simulink model "Sistema_LTI"  (R2016a)
settings: Solver=ode15s  StartTime=0.0  StopTime=5  RelTol=1e-3
PreLoadFcn:
  | parametros
values from neighbouring files (symbols this model uses):
  beq = (bm+bl/r^2)    (= 1.5637748692e-05)    [parametros.m]    (also in planificador_de_trayectoria.m)
  Jeq = (Jm+Jl/r^2)    (= 6.92649215207e-06)    [parametros.m]    (also in planificador_de_trayectoria.m)
  lambda_m = 0.01546    [parametros.m]
  Lq = 5.8e-3    (= 0.0058)    [parametros.m]
  Pp = 3    [parametros.m]
  r = 314.3008    [parametros.m]    (also in planificador_de_trayectoria.m)
  Rs = 1.02    [parametros.m]
settings Model: Creator=Jere  LastModifiedBy=Jere

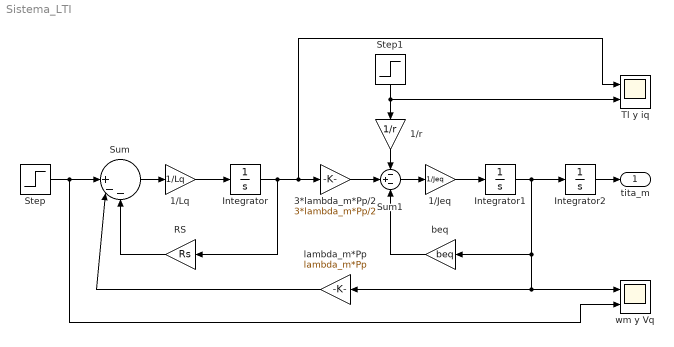
== system Sistema_LTI ==
  1/Jeq : Gain  Gain=1/Jeq
  1/Lq : Gain  Gain=1/Lq
  1/r : Gain  Gain=1/r
  3*lambda_m*Pp/2 : Gain  Gain=3*lambda_m*Pp/2
  Integrator : Integrator
  Integrator1 : Integrator
  Integrator2 : Integrator
  RS : Gain  Gain=Rs
  Step : Step  Time=0.1  After=19.596  SampleTime=0
  Step1 : Step  Time=0.3  After=1.57  SampleTime=0
  Sum : Sum  Inputs=||+--
  Sum1 : Sum  Inputs=-+-
  Tl y iq : Scope  NumInputPorts=2
  beq : Gain  Gain=beq
  lambda_m*Pp : Gain  Gain=lambda_m*Pp
  wm y Vq : Scope  NumInputPorts=2
  tita_m : Outport
  wires:
  Integrator/1 -> RS/1, Tl y iq/1, 3*lambda_m*Pp/2/1
  Integrator1/1 -> wm y Vq/1, lambda_m*Pp/1, beq/1, Integrator2/1
  Sum1/1 -> 1/Jeq/1
  1/r/1 -> Sum1/1
  3*lambda_m*Pp/2/1 -> Sum1/2
  RS/1 -> Sum/3
  Sum/1 -> 1/Lq/1
  1/Lq/1 -> Integrator/1
  beq/1 -> Sum1/3
  1/Jeq/1 -> Integrator1/1
  lambda_m*Pp/1 -> Sum/2
  Step/1 -> Sum/1, wm y Vq/2
  Step1/1 -> Tl y iq/2, 1/r/1
  Integrator2/1 -> tita_m/1
